simulink model "simu_21uec072"  (R2022b)
settings: Solver=VariableStepAuto  StartTime=0.0  StopTime=10.0  RelTol=1e-3
libraries: dspsnks4 x1, dspvision x1
settings Model: Creator=ECAD-17  LastModifiedBy=DSP-27

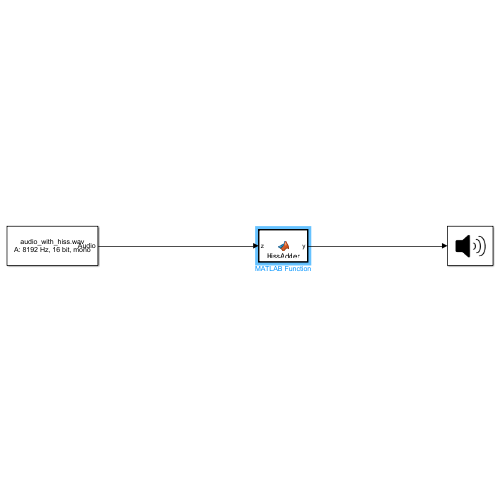
[thumbnail: Simulink's stored preview of the top-level diagram]
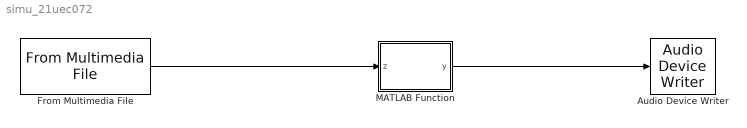
== system simu_21uec072 ==
  Audio Device Writer : dspsnks4/Audio Device Writer  Driver=DirectSound  Device=Default  InheritSampleRate=on  SampleRate=44100  BitDepth=16-bit integer  BufferSize=4096  NumBuffers=10  DefaultOutputChannelMapping=on  OutputChannelMapping=1:2  OutputNumUnderrunSamples=off  DriverIdx=1  DeviceWarnFlag=''
  From Multimedia File : dspvision/From Multimedia File  inputFilename=C:\Users\DSP-27\Desktop\21uec072\audio_with_hiss.wav  readRange=[1 Inf]  loop=on  numPlays=inf  outputStreams=Audio only  videoDataType=single  audioDataType=double  inheritSampleTime=on  userDefinedSampleTime=1/30  noAudioOutput=off  isIntensityVideo=off  fourcc=RGB  colorVideoFormat=Separate color signals  outputEOF=off  dataOrg=Column-major  audioFrameSize=256  computeAudioFrameSize=off  outSamplingMode=Sample based
      settings: LibrarySourceBlock=audiosources/From Multimedia File
  MATLAB Function : MATLAB Function  TreatAsAtomicUnit=on
  wires:
  From Multimedia File/1 -> MATLAB Function/1(z)
  MATLAB Function/1(y) -> Audio Device Writer/1

== matlab function simu_21uec072/MATLAB Function ==
  data: z input; y output
function y = convol(z)

h = [1, -2 * cos(pi/2), 1];
y1 = conv(z,h); 
y = y1;
